simulink model "Rail_TempLim"  (R2016b)
settings: configuration reference "CodeGenConfigSet" (kept outside this file)
values from neighbouring files (symbols this model uses):
  Rail_facFlPLimFTSCor_CUR = Calibration.Parameter    [init_Rail_TempLim.m]
  Rail_facFlPLimFTSCor_CURX = Calibration.Parameter    [init_Rail_TempLim.m]
  Rail_trqFlPLim_MAP = Calibration.Parameter    [init_Rail_TempLim.m]
  Rail_trqFlPLim_MAPX = Calibration.Parameter    [init_Rail_TempLim.m]
  Rail_trqFlPLim_MAPY = Calibration.Parameter    [init_Rail_TempLim.m]
  Rail_trqFlTempLimMeUn_MAP = Calibration.Parameter    [init_Rail_TempLim.m]
  Rail_trqFlTempLimMeUn_MAPX = Calibration.Parameter    [init_Rail_TempLim.m]
  Rail_trqFlTempLimMeUn_MAPY = Calibration.Parameter    [init_Rail_TempLim.m]
settings Model: Creator=lenovo  LastModifiedBy=wangrui
settings ConfigSetRef: SourceLocation=Base Workspace

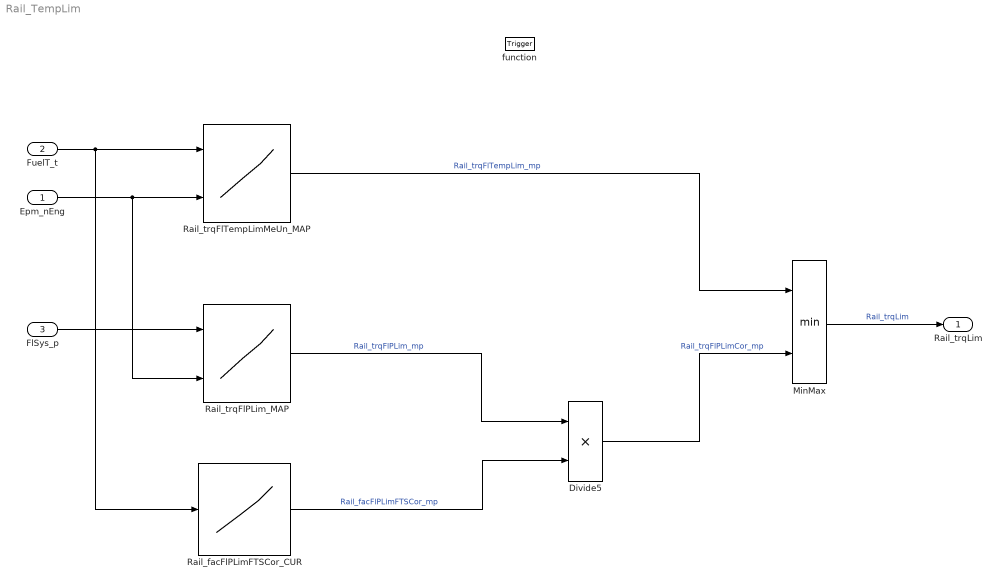
== system Rail_TempLim ==
  Epm_nEng : Inport  Tag=rpm  Description=Engine speed  OutMin=0  OutMax=6000  OutDataTypeStr=EngSpeed_rpm
  FuelT_t : Inport  Tag=deg  Description=Temperature of fuel  Port=2  OutMin=-50  OutMax=150  OutDataTypeStr=Temp_deg
  FlSys_p : Inport  Tag=kPa  Description=Fuelpressure on high pressure pump  Port=3  OutMin=0  OutMax=3000  OutDataTypeStr=AirPressure_kPa
  function : TriggerPort  TriggerType=function-call  VariantControl=Variant
  Divide5 : Product  Inputs=**  OutDataTypeStr=Trq_Nm
  MinMax : MinMax  Inputs=2  InputSameDT=on
  Rail_facFlPLimFTSCor_CUR : Lookup_n-D  NumberOfTableDimensions=1  BreakpointsForDimension1=Rail_facFlPLimFTSCor_CURX  IndexSearchMethod=Linear search  BeginIndexSearchUsingPreviousIndexResult=on  Table=Rail_facFlPLimFTSCor_CUR  ExtrapMethod=Clip  UseLastTableValue=on  InternalRulePriority=Speed  OutDataTypeStr=Inherit: Inherit via back propagation  SaturateOnIntegerOverflow=on
  Rail_trqFlPLim_MAP : Lookup_n-D  BreakpointsForDimension1=Rail_trqFlPLim_MAPY  BreakpointsForDimension2=Rail_trqFlPLim_MAPX  IndexSearchMethod=Linear search  BeginIndexSearchUsingPreviousIndexResult=on  Table=Rail_trqFlPLim_MAP  ExtrapMethod=Clip  UseLastTableValue=on  InternalRulePriority=Speed  OutDataTypeStr=Inherit: Inherit via back propagation  SaturateOnIntegerOverflow=on
  Rail_trqFlTempLimMeUn_MAP : Lookup_n-D  BreakpointsForDimension1=Rail_trqFlTempLimMeUn_MAPY  BreakpointsForDimension2=Rail_trqFlTempLimMeUn_MAPX  IndexSearchMethod=Linear search  BeginIndexSearchUsingPreviousIndexResult=on  Table=Rail_trqFlTempLimMeUn_MAP  ExtrapMethod=Clip  UseLastTableValue=on  InternalRulePriority=Speed  OutDataTypeStr=Inherit: Inherit via back propagation  SaturateOnIntegerOverflow=on
  Rail_trqLim : Outport  Tag=Nm  Description=Torque limitation dependent on fuel temperature  OutMin=0  OutMax=3000  OutDataTypeStr=Trq_Nm
  wires:
  FlSys_p/1 -> Rail_trqFlPLim_MAP/1
  MinMax/1 -> Rail_trqLim/1  "Rail_trqLim"
  Rail_trqFlTempLimMeUn_MAP/1 -> MinMax/1  "Rail_trqFlTempLim_mp"
  Rail_facFlPLimFTSCor_CUR/1 -> Divide5/2  "Rail_facFlPLimFTSCor_mp"
  Rail_trqFlPLim_MAP/1 -> Divide5/1  "Rail_trqFlPLim_mp"
  Divide5/1 -> MinMax/2  "Rail_trqFlPLimCor_mp"
  FuelT_t/1 -> Rail_trqFlTempLimMeUn_MAP/1, Rail_facFlPLimFTSCor_CUR/1
  Epm_nEng/1 -> Rail_trqFlTempLimMeUn_MAP/2, Rail_trqFlPLim_MAP/2
